simulink model "pipe_biflow_r01"  (R2018b)
settings: Solver=VariableStepAuto  StartTime=0.0  StopTime=24*3600  RelTol=1e-3
undefined symbols (not defined in the file): path_carnot
libraries: carnot x9, simulink x2
settings Model: Creator=drhf  LastModifiedBy=drhf

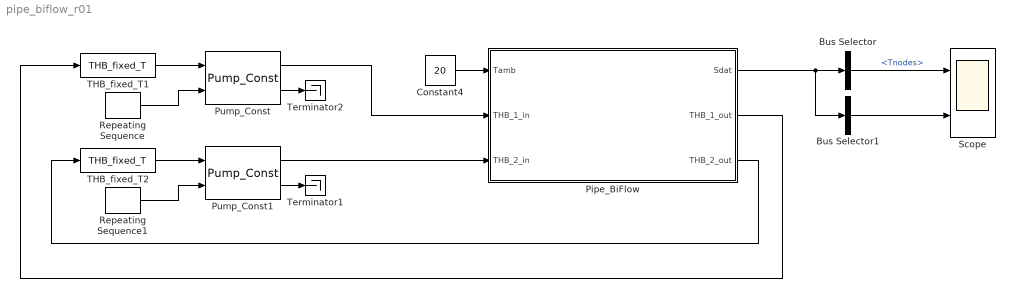
== system pipe_biflow_r01 ==
  Bus Selector : BusSelector  OutputSignals=Tnodes
  Bus Selector1 : BusSelector  OutputSignals=THBout_pipe1.MassFlow,THBin_pipe2.MassFlow  OutputAsBus=on
  Constant4 : Constant  Value=20
  Pipe_BiFlow : Subsystem  mask(Buffer storage tank){t0=20, hgt=1273.2395, stgtype=1, tini=[20 20 20 20 20 20 20 20 20 20], mpts=[1 2 3 4 5 6 7 8 9 10], PathName=fullfile(path_carnot('libsl'),'Storage','Thermal','Storage_Type_1','parameter_set'), FileName='<user defined>', userPath=off, userParam=on, uwall=1, ubot=1, utop=1, axcond=1, volume=10, dia=0.1, standing=standing cylinder, nodes=10, mpoints=10, pipe1inlet=1, pipe1outlet=0, pipe1dia=0.1, pipe2inlet=0, pipe2outlet=1, pipe2dia=0.1}
      mask prompts: t0 "Initial temperature (vector or scalar) in °C"; hgt "Height of storage in m"; stgtype "Storage Type (0..5)"; tini "Start temperatures of nodes in °C"; mpts "Index to measured nodes"; PathName "Path"; FileName "Parameter set"; userPath "Edit path and name of parameter set"; userParam "User defined parameters"; uwall "Heat transfer coefficient to ambient [W/m²K]"; ubot "Heat transfer coefficient to ambient bottom [W/m²K]"; utop "Heat transfer coefficient to ambient top [W/m²K]"; axcond "Effective thermal conductivity [W/m/K]"; volume "Volume [m³]"; dia "Diameter [m]"; standing "Position"; nodes "Number of nodes"; mpoints "Number of node temperatures (for display)"; pipe1inlet "relative height of inlet, range from 0 (= bottom) to 1 (= top)"; pipe1outlet "relative height of outlet, range from 0 (= bottom) to 1 (= top)"; pipe1dia "Diameter of pipe in m"; pipe2inlet "relative height of inlet, range from 0 (= bottom) to 1 (= top)"; pipe2outlet "relative height of outlet, range from 0 (= bottom) to 1 (= top)"; pipe2dia "Diameter of pipe in m"
      mask help:
      | Buffer storage for heating circuits. The storage model has the following components (with their typical position):
      | - one pipe connection for discharging (total height)
      | - one pipe connection for charging (total height)
      mask init:
      | [ok, param] = CarnotCallbacks_StorageConf('SetParam',stgtype,gcbh,PathName,FileName);
      mask Help: web(fullfile(path_carnot('help'),'Storage_Type_N.html'),'-helpbrowser')
      mask TypeOptions hgt: Pipe_Connection_1/hgt | Pipe_Connection_2/hgt
      mask TypeOptions stgtype: CreateSdat/stgtype
      mask TypeOptions tini: sfun_storageTnodes/tini
      mask TypeOptions mpts: select_T/Indices
      mask Callback userPath: [ok, param] = CarnotCallbacks_StorageConf('UserEdit',1,gcbh);
      mask Callback userParam: [ok, param] = CarnotCallbacks_StorageConf('UserEdit',1,gcbh);
      mask TypeOptions uwall: sfun_storageTnodes/uloss
      mask TypeOptions ubot: sfun_storageTnodes/ubot
      mask TypeOptions utop: sfun_storageTnodes/utop
      mask TypeOptions axcond: sfun_storageTnodes/cond
      mask TypeOptions volume: sfun_storageTnodes/volume | CreateSdat/volume
      mask TypeOptions dia: sfun_storageTnodes/dia | Pipe_Connection_1/dstg | Pipe_Connection_2/dstg
      mask TypeOptions standing: sfun_storageTnodes/standing
      mask TypeOptions nodes: sfun_storageTnodes/nodes | select_T/InputPortWidth | HX_EN12977_1/nodes | HX_EN12977_2/nodes | HX_EN12977_3/nodes | Pipe_Connection_1/nodes | Pipe_Connection_2/nodes | Pipe_Connection_3/nodes
      mask TypeOptions pipe1inlet: Pipe_Connection_1/h_in
      mask TypeOptions pipe1outlet: Pipe_Connection_1/h_out
      mask TypeOptions pipe1dia: Pipe_Connection_1/dpipe
      mask TypeOptions pipe2inlet: Pipe_Connection_2/h_in
      mask TypeOptions pipe2outlet: Pipe_Connection_2/h_out
      mask TypeOptions pipe2dia: Pipe_Connection_2/dpipe
      mask DialogControl Container14 Prompt: Infos
      mask DialogControl ParameterGroupVar Prompt: Picking a parameter set
      mask DialogControl Control3 Prompt: Carnot public data
      mask DialogControl Control3 Callback: [ok, file] = CarnotCallbacks_StorageConf('GetFilename',1,gcbh,'public');
      mask DialogControl Control4 Prompt: Carnot internal data
      mask DialogControl Control4 Callback: [ok, file] = CarnotCallbacks_StorageConf('GetFilename',1,gcbh,'internal');
      mask DialogControl Control2 Prompt: Selected path
      mask DialogControl Control2 Callback: [ok, file] = CarnotCallbacks_StorageConf('GetFilename',1,gcbh,'selected');
      mask DialogControl Container4 Prompt: Parameter values
      mask DialogControl Container6 Prompt: Storage
      mask DialogControl Container8 Prompt: Connections
      mask DialogControl Container9 Prompt: Charging pipe
      mask DialogControl Container12 Prompt: Discharging pipe
      mask DialogControl Control6 Prompt: Save in Carnot internal data
      mask DialogControl Control6 Callback: [ok, param] = CarnotCallbacks_StorageConf('SaveFilename',1,gcbh,'internal','STG');
      mask DialogControl Control5 Prompt: Save in selected path
      mask DialogControl Control5 Callback: [ok, param] = CarnotCallbacks_StorageConf('SaveFilename',1,gcbh,'selected','STG');
      mask Display:
      | % user defined picture file
      | namestr = ['Storage_Type_', num2str(get_param(gcb,'stgtype'))];
      | picfile = fullfile(path_carnot('intlibsl'), 'Storage','Thermal', ...
      |     namestr,'parameter_set', [namestr, '.jpg']);
      | 
      | % show internal picture if defined
      | pic = false;
      | if  ~BlockIsInCarnotLibrary       % if not located in library
      |     if exist(picfile, 'file')
      |         image(imread(picfile), [0.25, 0, 0.45, 1])
      |         set_param(gcb, 'BackgroundColor', 'White')
      |         pic = true;
      |     end
      | end
      | 
      | % show public picture
      | if ~pic
      |     set_param(gcb, 'BackgroundColor', 'Red')
      |     plot(0,0,1,1,[24,27,27,24,75,80,80,75,24,20,20,24]/100,[60,53,46,40,40,46,55,60,60,53,46,40]/100)
      | end
  Pump_Const : carnot/Hydraulics/Pump_Const  mdotmax=1800/3600  dia=0.02  p0=3e5  fluid_id=Water  mix=0  mix2=0  mix3=0  UA=3  mcp=4182  Tini=20  e0=10  e1=10  e2=-1
      settings: SourceProductName=Carnot
  Pump_Const1 : carnot/Hydraulics/Pump_Const  mdotmax=1200/3600  dia=0.02  p0=3e5  fluid_id=Water  mix=0  mix2=0  mix3=0  UA=3  mcp=4182  Tini=20  e0=10  e1=10  e2=-1
      settings: SourceProductName=Carnot
  Repeating Sequence : simulink/Sources/Repeating Sequence  rep_seq_t=[0 11.5 12.5 24]*3600  rep_seq_y=[1 1 0 0]
  Repeating Sequence1 : simulink/Sources/Repeating Sequence  rep_seq_t=[0 11.5 12.5 24]*3600  rep_seq_y=[0 0 1 1]
  Scope : Scope  NumInputPorts=2
  THB_fixed_T1 : carnot/Source/Simple/THB_fixed_T  t=60
      settings: SourceProductName=Carnot
  THB_fixed_T2 : carnot/Source/Simple/THB_fixed_T  t=40
      settings: SourceProductName=Carnot
  Terminator1 : Terminator
  Terminator2 : Terminator
  wires:
  THB_fixed_T1/1 -> Pump_Const/1
  Pump_Const/2 -> Terminator2/1
  Repeating Sequence/1 -> Pump_Const/2
  Constant4/1 -> Pipe_BiFlow/1(Tamb)
  Pipe_BiFlow/1(Sdat) -> Bus Selector1/1, Bus Selector/1
  Pump_Const/1 -> Pipe_BiFlow/2(THB_1_in)
  Pump_Const1/1 -> Pipe_BiFlow/3(THB_2_in)
  Repeating Sequence1/1 -> Pump_Const1/2
  Pump_Const1/2 -> Terminator1/1
  THB_fixed_T2/1 -> Pump_Const1/1
  Pipe_BiFlow/2(THB_1_out) -> THB_fixed_T1/1
  Pipe_BiFlow/3(THB_2_out) -> THB_fixed_T2/1
  Bus Selector/1 -> Scope/1  "<Tnodes>"
  Bus Selector1/1 -> Scope/2

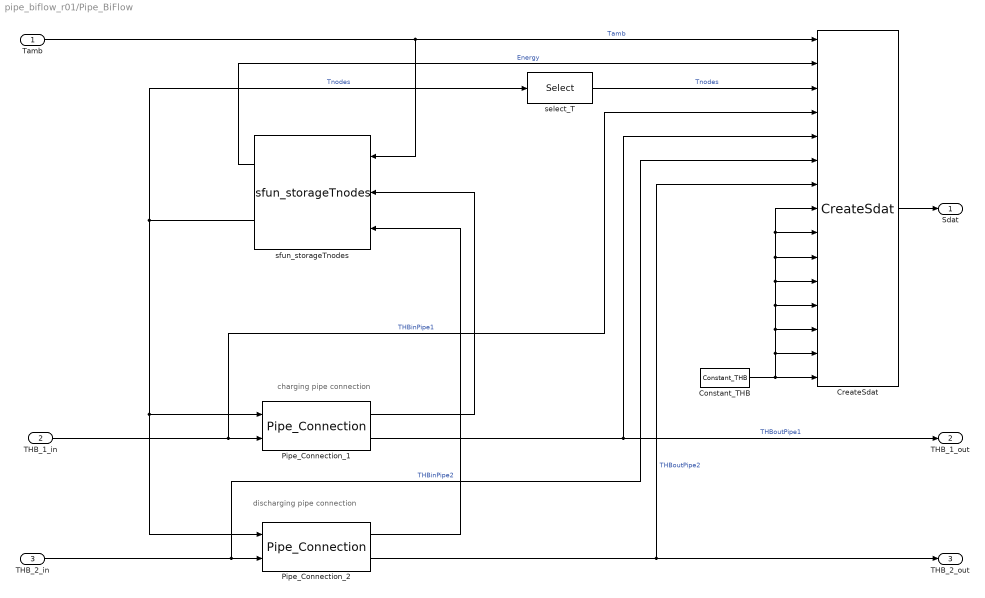
== system pipe_biflow_r01/Pipe_BiFlow ==
  note: discharging pipe connection
  note: charging pipe connection
  Tamb : Inport
  THB_1_in : Inport  Port=2
  THB_2_in : Inport  Port=3
  Constant_THB : carnot/Source/Simple/Constant_THB  t=20  mdot=0  p=1e5  mID=No Pressure Drop  fluid=Water  mix=0  mix2=0  mix3=0  dia=0.02  hgt=0
      settings: SourceProductName=Carnot
  CreateSdat : carnot/Basic/Thermal_Models/CreateSdat  volume=volume  stgtype=stgtype
      settings: SourceProductName=Carnot
  Pipe_Connection_1 : carnot/Storage/Thermal/Storage_Ports/Pipe_Connection  h_in=pipe1inlet  h_out=pipe1outlet  hgt=hgt  dpipe=pipe1dia  dstg=dia  height=-1273.2395  nodes=nodes
      settings: SourceProductName=Carnot
  Pipe_Connection_2 : carnot/Storage/Thermal/Storage_Ports/Pipe_Connection  h_in=pipe2inlet  h_out=pipe2outlet  hgt=hgt  dpipe=pipe2dia  dstg=dia  height=1273.2395  nodes=nodes
      settings: SourceProductName=Carnot
  select_T : Selector  InputPortWidth=nodes  IndexOptions=Index vector (dialog)  Indices=[1 2 3 4 5 6 7 8 9 10]  OutputSizes=1
  sfun_storageTnodes : carnot/Basic/Thermal_Models/sfun_storageTnodes  uloss=uwall  ubot=ubot  utop=utop  cond=axcond  volume=volume  dia=dia  standing=standing cylinder  tini=tini  nodes=nodes  nconnect=2  elimthermocline=0  condinvtc=0
      settings: SourceProductName=Carnot
  Sdat : Outport
  THB_1_out : Outport  Port=2
  THB_2_out : Outport  Port=3
  wires:
  Constant_THB/1 -> CreateSdat/15, CreateSdat/8, CreateSdat/9, CreateSdat/10, CreateSdat/11, CreateSdat/12, CreateSdat/13, CreateSdat/14
  Pipe_Connection_1/1 -> sfun_storageTnodes/2
  Pipe_Connection_1/2 -> THB_1_out/1, CreateSdat/5  "THBoutPipe1"
  THB_1_in/1 -> Pipe_Connection_1/2, CreateSdat/4  "THBinPipe1"
  CreateSdat/1 -> Sdat/1
  sfun_storageTnodes/2 -> select_T/1, Pipe_Connection_1/1, Pipe_Connection_2/1  "Tnodes"
  select_T/1 -> CreateSdat/3  "Tnodes"
  Tamb/1 -> CreateSdat/1, sfun_storageTnodes/1  "Tamb"
  THB_2_in/1 -> CreateSdat/6, Pipe_Connection_2/2  "THBinPipe2"
  Pipe_Connection_2/1 -> sfun_storageTnodes/3
  Pipe_Connection_2/2 -> THB_2_out/1, CreateSdat/7  "THBoutPipe2"
  sfun_storageTnodes/1 -> CreateSdat/2  "Energy"
